simulink model "ccpi"  (R2021b)
settings: Solver=VariableStepAuto  StartTime=0.0  StopTime=10.0  RelTol=1e-3
undefined symbols (not defined in the file): b, Ki, Kp, m
settings Model: Creator=feyzi  LastModifiedBy=feyzi

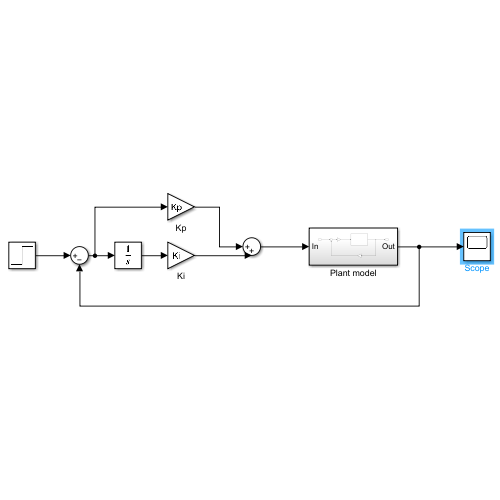
[thumbnail: Simulink's stored preview of the top-level diagram]
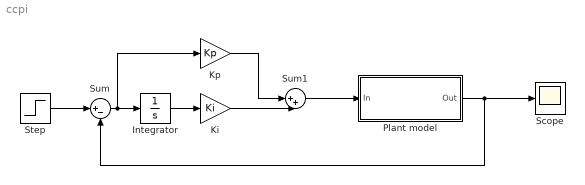
== system ccpi ==
  Integrator : Integrator
  Ki : Gain  Gain=Ki
  Kp : Gain  Gain=Kp
  Plant model : Subsystem
  Scope : Scope
  Step : Step  Time=0  After=u  SampleTime=0
  Sum : Sum  Inputs=|+-
  Sum1 : Sum  Inputs=|++
  wires:
  Plant model/1(Out) -> Scope/1, Sum/2
  Sum/1 -> Kp/1, Integrator/1
  Integrator/1 -> Ki/1
  Ki/1 -> Sum1/2
  Kp/1 -> Sum1/1
  Sum1/1 -> Plant model/1(In)
  Step/1 -> Sum/1

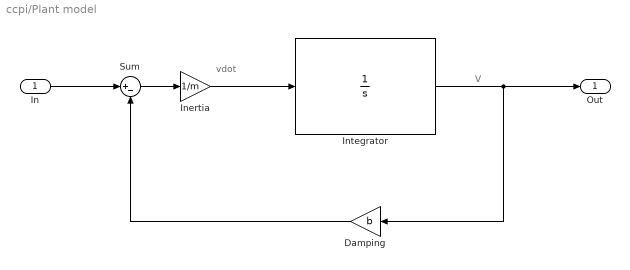
== system ccpi/Plant model ==
  note: V
  note: vdot
  In : Inport
  Damping : Gain  Gain=b
  Inertia : Gain  Gain=1/m
  Integrator : Integrator  ContinuousStateAttributes="\"Integrator\""
  Sum : Sum  Inputs=|+-
  Out : Outport
  wires:
  Damping/1 -> Sum/2
  Integrator/1 -> Out/1, Damping/1
  In/1 -> Sum/1
  Inertia/1 -> Integrator/1
  Sum/1 -> Inertia/1
